simulink model "transfer_function_model"  (R2016a)
settings: Solver=VariableStepAuto  StartTime=0.0  StopTime=100  RelTol=1e-3
settings Model: Creator=mikae  LastModifiedBy=mikae

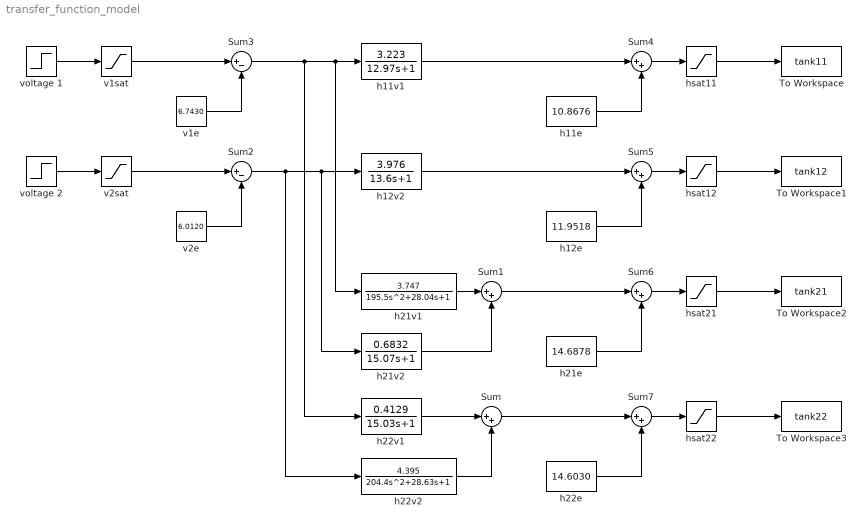
== system transfer_function_model ==
  Sum{,1,4..7} (6 alike) : Sum  Inputs=|++
  Sum2 : Sum  Inputs=|+-
  Sum3 : Sum  Inputs=|+-
  To Workspace : ToWorkspace  VariableName=tank11  SaveFormat=Timeseries  SampleTime=-1
  To Workspace1 : ToWorkspace  VariableName=tank12  SaveFormat=Timeseries  SampleTime=-1
  To Workspace2 : ToWorkspace  VariableName=tank21  SaveFormat=Timeseries  SampleTime=-1
  To Workspace3 : ToWorkspace  VariableName=tank22  SaveFormat=Timeseries  SampleTime=-1
  h11e : Constant  Value=10.8676
  h11v1 : TransferFcn  Numerator=[3.223]  Denominator=[12.97 1]
  h12e : Constant  Value=11.9518
  h12v2 : TransferFcn  Numerator=[3.976]  Denominator=[13.6 1]
  h21e : Constant  Value=14.6878
  h21v1 : TransferFcn  Numerator=[3.747]  Denominator=[195.5 28.04 1]
  h21v2 : TransferFcn  Numerator=[0.6832]  Denominator=[15.07 1]
  h22e : Constant  Value=14.6030
  h22v1 : TransferFcn  Numerator=[0.4129]  Denominator=[15.03 1]
  h22v2 : TransferFcn  Numerator=[4.395]  Denominator=[204.4 28.63 1]
  hsat{11..12,21..22} (4 alike) : Saturate  UpperLimit=30  LowerLimit=0
  v1e : Constant  Value=6.7430
  v1sat : Saturate  UpperLimit=12  LowerLimit=0
  v2e : Constant  Value=6.0120
  v2sat : Saturate  UpperLimit=12  LowerLimit=0
  voltage 1 : Step  Time=30  After=6.7430  SampleTime=0
  voltage 2 : Step  Time=30  After=6.0120  SampleTime=0
  wires:
  hsat12/1 -> To Workspace1/1
  hsat21/1 -> To Workspace2/1
  hsat22/1 -> To Workspace3/1
  voltage 1/1 -> v1sat/1
  voltage 2/1 -> v2sat/1
  h21v1/1 -> Sum1/1
  h21v2/1 -> Sum1/2
  h22v1/1 -> Sum/1
  h22v2/1 -> Sum/2
  h11v1/1 -> Sum4/1
  Sum5/1 -> hsat12/1
  h12v2/1 -> Sum5/1
  Sum1/1 -> Sum6/1
  Sum6/1 -> hsat21/1
  Sum/1 -> Sum7/1
  Sum7/1 -> hsat22/1
  v1sat/1 -> Sum3/1
  v2sat/1 -> Sum2/1
  Sum3/1 -> h22v1/1, h21v1/1, h11v1/1
  Sum2/1 -> h22v2/1, h21v2/1, h12v2/1
  h11e/1 -> Sum4/2
  h12e/1 -> Sum5/2
  h21e/1 -> Sum6/2
  h22e/1 -> Sum7/2
  v1e/1 -> Sum3/2
  v2e/1 -> Sum2/2
  hsat11/1 -> To Workspace/1
  Sum4/1 -> hsat11/1
